simulink model "Ej_Voz"  (Simulink 8.6)
settings: Solver=VariableStepAuto  StartTime=0.0  StopTime=50.0  FixedStep=1/22050  RelTol=1e-3
undefined symbols (not defined in the file or in its folder): Fs, get
libraries: dspsnks4 x2, dspsrcs4 x1, dspspect3 x1
settings Model: Creator=Milton  LastModifiedBy=fernando
settings DebuggingCC: FcnCallInpInsideContextMsg=UseLocalSettings
settings HardwareCC: ProdIntDivRoundTo=Zero  ProdEndianess=LittleEndian  ProdHWDeviceType=Custom Processor->Custom

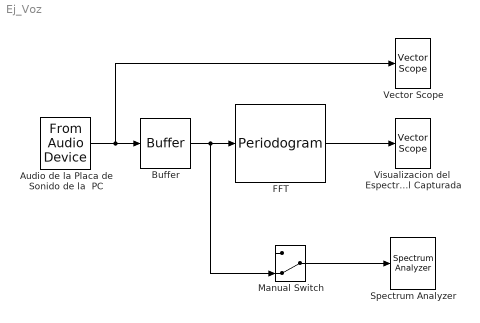
== system Ej_Voz ==
  Audio de la Placa de Sonido de la  PC : dspsrcs4/From Audio Device  deviceName=Default  numChannels=1  sampleRate=22050  deviceDatatype=24-bit integer  autoBufferSize=on  bufferSize=4096  queueDuration=10  frameSize=512  outputDatatype=double  defaultInputChannelMapping=on  inputChannelMapping=1:2  outputNumOverrunSamples=off  OutputFrames=on
  Buffer : Buffer  N=2048  V=48
  FFT : dspspect3/Periodogram  measurement=Mean-square spectrum  wintype=Hamming  Rs=50  beta=5  winsamp=Periodic  FFTImplementation=Auto  inheritFFT=on  fftsize=512  navg=2  inheritTs=on  Ts=1
  Manual Switch : ManualSwitch  CurrentSetting=0
  Spectrum Analyzer : SpectrumAnalyzer
  Vector Scope : dspsnks4/Vector Scope  ScopeProperties=on  Domain=Time  HorizSpan=1  DisplayProperties=off  AxisGrid=on  Memory=off  FrameNumber=on  AxisLegend=off  AxisZoom=off  OpenScopeAtSimStart=on  OpenScopeImmediately=off  FigPos=get(0,'defaultfigureposition')  AxisProperties=off  XUnits=Hertz  XRange=[0...Fs/2]  InheritXIncr=on  XIncr=1  XLabel=Time  XLimit=Auto  XMin=0  XMax=1  XStart=0  YUnits=dB  YLabel=Amplitude  LineProperties=off  XAxisParamsVer=6.9
      settings: YMin=-1  YMax=1
  Visualizacion del  Espectro de la Señal Capturada : dspsnks4/Vector Scope  ScopeProperties=off  Domain=Frequency  HorizSpan=1  DisplayProperties=on  AxisGrid=on  Memory=off  FrameNumber=off  AxisLegend=off  AxisZoom=off  OpenScopeAtSimStart=on  OpenScopeImmediately=off  FigPos=[80 110 380 320]  AxisProperties=off  XUnits=Hertz  XRange=[-Fs/2...Fs/2]  InheritXIncr=on  XIncr=1  XLabel=Samples  XLimit=User-defined  XMin=0  XMax=11567.2131  XStart=0  YUnits=dB  YLabel=Magnitude, dB  LineProperties=off  XAxisParamsVer=6.9
      settings: YMin=-170  YMax=-30
  wires:
  FFT/1 -> Visualizacion del  Espectro de la Señal Capturada/1
  Audio de la Placa de Sonido de la  PC/1 -> Buffer/1, Vector Scope/1
  Buffer/1 -> Manual Switch/2, FFT/1
  Manual Switch/1 -> Spectrum Analyzer/1
